simulink library "SIMULINK_PS_LIB"  (R2016b)
settings: Solver=VariableStepAuto  StartTime=0.0  StopTime=10.0  RelTol=1e-3
libraries: nesl_utility x1
settings Model: Creator=IFO37  LastModifiedBy=IFO37

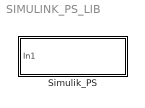
== system SIMULINK_PS_LIB ==
  Simulik_PS : Subsystem

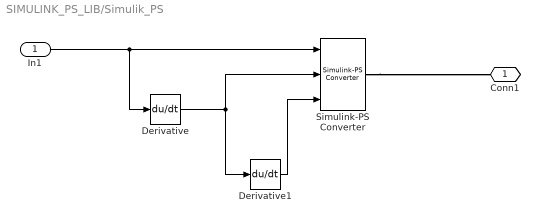
== system SIMULINK_PS_LIB/Simulik_PS ==
  In1 : Inport
  Derivative : Derivative
  Derivative1 : Derivative
  Simulink-PS Converter : nesl_utility/Simulink-PS Converter  PhysicalDomain=network_engine_domain  SubClassName=ps_input  LeftPortType=input  RightPortType=output  PseudoPeriodic=off  Frequencies=[]  NoiseDistribution=none  NoiseParameters=[]  Unit=1  AffineConversion=off  InputFiltering=derivs  SimscapeFilterOrder=1  InputFilterTimeConstant=0.001  UdotUserProvided=2
  Conn1 : PMIOPort  Port=1  Side=Right
  wires:
  Derivative1/1 -> Simulink-PS Converter/3
  Derivative/1 -> Simulink-PS Converter/2, Derivative1/1
  In1/1 -> Derivative/1, Simulink-PS Converter/1
  connections:
  Simulink-PS Converter/RConn1 -- Conn1/RConn1
